simulink model "comedi_linux_ert_test"  (R2013a)
settings: Solver=FixedStepDiscrete  StartTime=0.0  StopTime=inf  FixedStep=0.01  RelTol=1e-3
libraries: comedi_lib x9
settings Model: SimulationMode=external  Creator=pi  LastModifiedBy=pi
settings OptimizationCC: OptimizeModelRefInitCode=on  LifeSpan=Inf
settings RTWCC: SystemTargetFile=ert_linux.tlc  MakeCommand="make_rtw OPT_OPTS=\"-O2 -ggdb -Wall\" ADDITIONAL_LDFLAGS=\"-lcomedi\""  TemplateMakefile=ert_linux.tmf  Description=Linux Embedded Coder  ProcessScript=ert_linux_make_rtw_hook  CustomSource=comedi_lib.c  CheckMdlBeforeBuild=Warning
settings CodeAppCC: IgnoreCustomStorageClasses=off
settings STFCustomTargetCC: CodeReplacementLibrary=C99 (ISO)  ModelReferenceCompliant=off  CombineOutputUpdateFcns=on  ERTCustomFileBanners=on  SupportContinuousTime=off  MATLABClassNameForMDSCustomization=Simulink.SoftwareTarget.ERTCustomization  SystemTargetFile=ert_linux.tlc
settings ERTTargetCC: CodeReplacementLibrary=C99 (ISO)  GenerateSampleERTMain=off  ModelReferenceCompliant=off  ParMdlRefBuildCompliant=off  CompOptLevelCompliant=off  ConcurrentExecutionCompliant=off  ERTFirstTimeCompliant=off  SupportNonInlinedSFcns=on  ModelStepFunctionPrototypeControlCompliant=off  CPPClassGenCompliant=off  ExtMode=on  ERTCustomFileTemplate=ert_linux_file_process.tlc

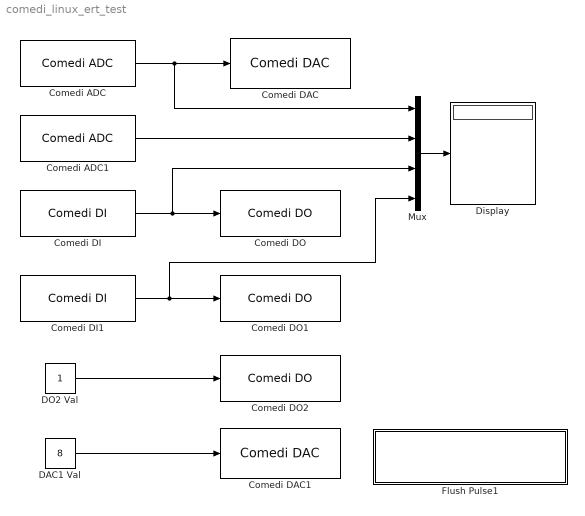
== system comedi_linux_ert_test ==
  Comedi ADC : comedi_lib/Comedi ADC  dev=comedi0  chan=0  range=0  aref=ground  dt=0.01
  Comedi ADC1 : comedi_lib/Comedi ADC  dev=comedi0  chan=1  range=0  aref=ground  dt=0.01
  Comedi DAC : comedi_lib/Comedi DAC  dev=comedi0  chan=0  range=0  aref=ground
  Comedi DAC1 : comedi_lib/Comedi DAC  dev=comedi0  chan=1  range=0  aref=ground
  Comedi DI : comedi_lib/Comedi DI  dev=comedi0  chan=0  dt=0.01
  Comedi DI1 : comedi_lib/Comedi DI  dev=comedi0  chan=1  dt=0.01
  Comedi DO : comedi_lib/Comedi DO  dev=comedi0  chan=0  threshold=0.5
  Comedi DO1 : comedi_lib/Comedi DO  dev=comedi0  chan=1  threshold=0.5
  Comedi DO2 : comedi_lib/Comedi DO  dev=comedi0  chan=2  threshold=0.5
  DAC1 Val : Constant  Value=8
  DO2 Val : Constant
  Display : Display
  Flush Pulse1 : Subsystem  mask{target_ip_address=''}
      mask prompts: target_ip_address "Target IP address"
      settings: OpenFcn=system(['./run_model.sh ', get_param(bdroot(gcbh),'name'),' ', get_param(gcbh,'target_ip_address')]);
      mask Display: disp('Double Click\n to run model\n(can select target IP)')
  Mux : Mux
  wires:
  Comedi ADC/1 -> Mux/1, Comedi DAC/1
  Comedi DI1/1 -> Mux/4, Comedi DO1/1
  Comedi DI/1 -> Mux/3, Comedi DO/1
  Mux/1 -> Display/1
  DAC1 Val/1 -> Comedi DAC1/1
  DO2 Val/1 -> Comedi DO2/1
  Comedi ADC1/1 -> Mux/2

== system comedi_linux_ert_test/Flush Pulse1 ==
